simulink model "IEEE9_case"  (R2024b)
settings: Solver=FixedStepAuto  StartTime=0  StopTime=5  FixedStep=1e-7  RelTol=1e-3
values from neighbouring files (symbols this model uses):
  SG_D_1_D = 0.01056    [IEEE9_case_parameters.m]    (also in case1_parameters.m; case2_parameters.m; case3_parameters.m; case4_parameters.m)
  SG_D_1_EnableSaturation = 0    [IEEE9_case_parameters.m]    (also in case1_parameters.m; case2_parameters.m; case3_parameters.m; case4_parameters.m)
  SG_D_1_f0 = 60    [IEEE9_case_parameters.m]    (also in case1_parameters.m; case2_parameters.m; case3_parameters.m; case4_parameters.m)
  SG_D_1_H = 7.5    [IEEE9_case_parameters.m]    (also in case1_parameters.m; case2_parameters.m; case3_parameters.m; case4_parameters.m)
  SG_D_1_K_A = 20    [IEEE9_case_parameters.m]    (also in case1_parameters.m; case2_parameters.m; case3_parameters.m; case4_parameters.m)
  SG_D_1_K_E = 1.000000e+1    (= 10)    [IEEE9_case_parameters.m]    (also in case1_parameters.m; case2_parameters.m; case3_parameters.m; case4_parameters.m)
  SG_D_1_K_F = 2.363    [IEEE9_case_parameters.m]    (also in case1_parameters.m; case2_parameters.m; case3_parameters.m; case4_parameters.m)
  SG_D_1_K_s = 0.5    [IEEE9_case_parameters.m]    (also in case1_parameters.m = 5; case2_parameters.m = 5; case3_parameters.m = 5; case4_parameters.m = 5)
  SG_D_1_R_a = 0.001088    [IEEE9_case_parameters.m]    (also in case1_parameters.m; case2_parameters.m; case3_parameters.m; case4_parameters.m)
  SG_D_1_S_A = 1    [IEEE9_case_parameters.m]    (also in case1_parameters.m; case2_parameters.m; case3_parameters.m; case4_parameters.m)
  SG_D_1_S_B = 0.103    [IEEE9_case_parameters.m]    (also in case1_parameters.m; case2_parameters.m; case3_parameters.m; case4_parameters.m)
  SG_D_1_S_N = 10.659857    [IEEE9_case_parameters.m]    (also in case1_parameters.m; case2_parameters.m; case3_parameters.m; case4_parameters.m)
  SG_D_1_SpeedPara = 200    [IEEE9_case_parameters.m]    (also in case1_parameters.m; case2_parameters.m; case3_parameters.m; case4_parameters.m)
  SG_D_1_T_0 = 0.720173    [IEEE9_case_parameters.m]    (also in case1_parameters.m = 0.755522; case2_parameters.m = 0.808931; case3_parameters.m = 0.869402; case4_parameters.m = 0.729316)
  SG_D_1_T_1 = 0.3    [IEEE9_case_parameters.m]    (also in case1_parameters.m; case2_parameters.m; case3_parameters.m; case4_parameters.m)
  SG_D_1_T_2 = 0.05    [IEEE9_case_parameters.m]    (also in case1_parameters.m; case2_parameters.m; case3_parameters.m; case4_parameters.m)
  SG_D_1_T_3 = 0.02    [IEEE9_case_parameters.m]    (also in case1_parameters.m; case2_parameters.m; case3_parameters.m; case4_parameters.m)
  SG_D_1_T_4 = 0.005    [IEEE9_case_parameters.m]    (also in case1_parameters.m; case2_parameters.m; case3_parameters.m; case4_parameters.m)
  SG_D_1_T_A = 0.02    [IEEE9_case_parameters.m]    (also in case1_parameters.m; case2_parameters.m; case3_parameters.m; case4_parameters.m)
  SG_D_1_T_dd = 8.000000e+0    (= 8)    [IEEE9_case_parameters.m]    (also in case1_parameters.m; case2_parameters.m; case3_parameters.m; case4_parameters.m)
  SG_D_1_T_ddd = 0.04    [IEEE9_case_parameters.m]    (also in case1_parameters.m; case2_parameters.m; case3_parameters.m; case4_parameters.m)
  SG_D_1_T_E = 0.314    [IEEE9_case_parameters.m]    (also in case1_parameters.m; case2_parameters.m; case3_parameters.m; case4_parameters.m)
  SG_D_1_T_F = 0.35    [IEEE9_case_parameters.m]    (also in case1_parameters.m; case2_parameters.m; case3_parameters.m; case4_parameters.m)
  SG_D_1_T_qd = 0.8    [IEEE9_case_parameters.m]    (also in case1_parameters.m; case2_parameters.m; case3_parameters.m; case4_parameters.m)
  SG_D_1_T_qdd = 0.02    [IEEE9_case_parameters.m]    (also in case1_parameters.m; case2_parameters.m; case3_parameters.m; case4_parameters.m)
  SG_D_1_T_speed = 0.1    [IEEE9_case_parameters.m]    (also in case1_parameters.m = 200; case2_parameters.m = 200; case3_parameters.m = 200; case4_parameters.m = 200)
  SG_D_1_T_w = 0.5    [IEEE9_case_parameters.m]    (also in case1_parameters.m; case2_parameters.m; case3_parameters.m; case4_parameters.m)
  SG_D_1_V_ref = 1.990276    [IEEE9_case_parameters.m]    (also in case1_parameters.m = 2.042296; case2_parameters.m = 2.051388; case3_parameters.m = 2.089584; case4_parameters.m = 2.01845)
  SG_D_1_w_ref = 376.991118    [IEEE9_case_parameters.m]    (also in case1_parameters.m; case2_parameters.m; case3_parameters.m; case4_parameters.m)
  SG_D_1_wb = 6.000000e+1    (= 60)    [IEEE9_case_parameters.m]    (also in case1_parameters.m; case2_parameters.m; case3_parameters.m; case4_parameters.m)
  SG_D_1_x_d = 1.9    [IEEE9_case_parameters.m]    (also in case1_parameters.m; case2_parameters.m; case3_parameters.m; case4_parameters.m)
  SG_D_1_x_dd = 0.302    [IEEE9_case_parameters.m]    (also in case1_parameters.m; case2_parameters.m; case3_parameters.m; case4_parameters.m)
  SG_D_1_x_ddd = 0.204    [IEEE9_case_parameters.m]    (also in case1_parameters.m; case2_parameters.m; case3_parameters.m; case4_parameters.m)
  SG_D_1_x_l = 0.05    [IEEE9_case_parameters.m]    (also in case1_parameters.m; case2_parameters.m; case3_parameters.m; case4_parameters.m)
  SG_D_1_x_q = 1.3    [IEEE9_case_parameters.m]    (also in case1_parameters.m; case2_parameters.m; case3_parameters.m; case4_parameters.m)
  SG_D_1_x_qd = 0.5    [IEEE9_case_parameters.m]    (also in case1_parameters.m; case2_parameters.m; case3_parameters.m; case4_parameters.m)
  SG_D_1_x_qdd = 0.3    [IEEE9_case_parameters.m]    (also in case1_parameters.m; case2_parameters.m; case3_parameters.m; case4_parameters.m)
  SG_D_2_D = 0.02    [IEEE9_case_parameters.m]    (also in case1_parameters.m; case2_parameters.m; case3_parameters.m; case4_parameters.m)
  SG_D_2_EnableSaturation = 0    [IEEE9_case_parameters.m]    (also in case1_parameters.m; case2_parameters.m; case3_parameters.m; case4_parameters.m)
  SG_D_2_f0 = 60    [IEEE9_case_parameters.m]    (also in case1_parameters.m; case2_parameters.m; case3_parameters.m; case4_parameters.m)
  SG_D_2_H = 8.000000e+0    (= 8)    [IEEE9_case_parameters.m]    (also in case1_parameters.m; case2_parameters.m; case3_parameters.m; case4_parameters.m)
  SG_D_2_K_A = 20    [IEEE9_case_parameters.m]    (also in case1_parameters.m; case2_parameters.m; case3_parameters.m; case4_parameters.m)
  SG_D_2_K_E = 1.000000e+1    (= 10)    [IEEE9_case_parameters.m]    (also in case1_parameters.m; case2_parameters.m; case3_parameters.m; case4_parameters.m)
  SG_D_2_K_F = 2.363    [IEEE9_case_parameters.m]    (also in case1_parameters.m; case2_parameters.m; case3_parameters.m; case4_parameters.m)
  SG_D_2_K_s = 0.5    [IEEE9_case_parameters.m]    (also in case1_parameters.m = 4; case2_parameters.m = 4; case3_parameters.m = 4; case4_parameters.m = 4)
  SG_D_2_R_a = 0.001088    [IEEE9_case_parameters.m]    (also in case1_parameters.m; case2_parameters.m; case3_parameters.m; case4_parameters.m)
  SG_D_2_S_A = 1    [IEEE9_case_parameters.m]    (also in case1_parameters.m; case2_parameters.m; case3_parameters.m; case4_parameters.m)
  SG_D_2_S_B = 0.103    [IEEE9_case_parameters.m]    (also in case1_parameters.m; case2_parameters.m; case3_parameters.m; case4_parameters.m)
  SG_D_2_S_N = 10.659857    [IEEE9_case_parameters.m]    (also in case1_parameters.m; case2_parameters.m; case3_parameters.m; case4_parameters.m)
  SG_D_2_SpeedPara = 200    [IEEE9_case_parameters.m]    (also in case1_parameters.m; case2_parameters.m; case3_parameters.m; case4_parameters.m)
  SG_D_2_T_0 = 1.632913    [IEEE9_case_parameters.m]    (also in case1_parameters.m = 1.632925; case2_parameters.m = 1.632915; case3_parameters.m = 1.632914; case4_parameters.m = 1.632927)
  SG_D_2_T_1 = 0.2    [IEEE9_case_parameters.m]    (also in case1_parameters.m; case2_parameters.m; case3_parameters.m; case4_parameters.m)
  SG_D_2_T_2 = 0.05    [IEEE9_case_parameters.m]    (also in case1_parameters.m; case2_parameters.m; case3_parameters.m; case4_parameters.m)
  SG_D_2_T_3 = 0.02    [IEEE9_case_parameters.m]    (also in case1_parameters.m; case2_parameters.m; case3_parameters.m; case4_parameters.m)
  SG_D_2_T_4 = 0.005    [IEEE9_case_parameters.m]    (also in case1_parameters.m; case2_parameters.m; case3_parameters.m; case4_parameters.m)
  SG_D_2_T_A = 0.02    [IEEE9_case_parameters.m]    (also in case1_parameters.m; case2_parameters.m; case3_parameters.m; case4_parameters.m)
  SG_D_2_T_dd = 7.9    [IEEE9_case_parameters.m]    (also in case1_parameters.m; case2_parameters.m; case3_parameters.m; case4_parameters.m)
  SG_D_2_T_ddd = 0.04    [IEEE9_case_parameters.m]    (also in case1_parameters.m; case2_parameters.m; case3_parameters.m; case4_parameters.m)
  SG_D_2_T_E = 0.314    [IEEE9_case_parameters.m]    (also in case1_parameters.m; case2_parameters.m; case3_parameters.m; case4_parameters.m)
  SG_D_2_T_F = 0.35    [IEEE9_case_parameters.m]    (also in case1_parameters.m; case2_parameters.m; case3_parameters.m; case4_parameters.m)
  SG_D_2_T_qd = 0.8    [IEEE9_case_parameters.m]    (also in case1_parameters.m; case2_parameters.m; case3_parameters.m; case4_parameters.m)
  SG_D_2_T_qdd = 0.015    [IEEE9_case_parameters.m]    (also in case1_parameters.m; case2_parameters.m; case3_parameters.m; case4_parameters.m)
  SG_D_2_T_speed = 0.1    [IEEE9_case_parameters.m]    (also in case1_parameters.m = 150; case2_parameters.m = 150; case3_parameters.m = 150; case4_parameters.m = 150)
  SG_D_2_T_w = 0.35    [IEEE9_case_parameters.m]    (also in case1_parameters.m; case2_parameters.m; case3_parameters.m; case4_parameters.m)
  SG_D_2_V_ref = 2.58547    [IEEE9_case_parameters.m]    (also in case1_parameters.m = 2.597896; case2_parameters.m = 2.587136; case3_parameters.m = 2.586042; case4_parameters.m = 2.599679)
  SG_D_2_w_ref = 376.991118    [IEEE9_case_parameters.m]    (also in case1_parameters.m; case2_parameters.m; case3_parameters.m; case4_parameters.m)
  SG_D_2_wb = 6.000000e+1    (= 60)    [IEEE9_case_parameters.m]    (also in case1_parameters.m; case2_parameters.m; case3_parameters.m; case4_parameters.m)
  SG_D_2_x_d = 1.8    [IEEE9_case_parameters.m]    (also in case1_parameters.m; case2_parameters.m; case3_parameters.m; case4_parameters.m)
  SG_D_2_x_dd = 0.302    [IEEE9_case_parameters.m]    (also in case1_parameters.m; case2_parameters.m; case3_parameters.m; case4_parameters.m)
  SG_D_2_x_ddd = 0.204    [IEEE9_case_parameters.m]    (also in case1_parameters.m; case2_parameters.m; case3_parameters.m; case4_parameters.m)
  SG_D_2_x_l = 0.05    [IEEE9_case_parameters.m]    (also in case1_parameters.m; case2_parameters.m; case3_parameters.m; case4_parameters.m)
  SG_D_2_x_q = 1.25    [IEEE9_case_parameters.m]    (also in case1_parameters.m; case2_parameters.m; case3_parameters.m; case4_parameters.m)
  SG_D_2_x_qd = 0.5    [IEEE9_case_parameters.m]    (also in case1_parameters.m; case2_parameters.m; case3_parameters.m; case4_parameters.m)
  SG_D_2_x_qdd = 0.3    [IEEE9_case_parameters.m]    (also in case1_parameters.m; case2_parameters.m; case3_parameters.m; case4_parameters.m)
  SG_D_3_D = 0.02    [IEEE9_case_parameters.m]    (also in case1_parameters.m; case2_parameters.m; case3_parameters.m; case4_parameters.m)
  SG_D_3_EnableSaturation = 0    [IEEE9_case_parameters.m]    (also in case1_parameters.m; case2_parameters.m; case3_parameters.m; case4_parameters.m)
  SG_D_3_f0 = 60    [IEEE9_case_parameters.m]    (also in case1_parameters.m; case2_parameters.m; case3_parameters.m; case4_parameters.m)
  SG_D_3_H = 7.7    [IEEE9_case_parameters.m]    (also in case1_parameters.m; case2_parameters.m; case3_parameters.m; case4_parameters.m)
  SG_D_3_K_A = 20    [IEEE9_case_parameters.m]    (also in case1_parameters.m; case2_parameters.m; case3_parameters.m; case4_parameters.m)
  SG_D_3_K_E = 1.000000e+1    (= 10)    [IEEE9_case_parameters.m]    (also in case1_parameters.m; case2_parameters.m; case3_parameters.m; case4_parameters.m)
  SG_D_3_K_F = 2.363    [IEEE9_case_parameters.m]    (also in case1_parameters.m; case2_parameters.m; case3_parameters.m; case4_parameters.m)
  SG_D_3_K_s = 0.2    [IEEE9_case_parameters.m]    (also in case1_parameters.m = 2; case2_parameters.m = 2; case3_parameters.m = 2; case4_parameters.m = 2)
  SG_D_3_R_a = 0.001088    [IEEE9_case_parameters.m]    (also in case1_parameters.m; case2_parameters.m; case3_parameters.m; case4_parameters.m)
  SG_D_3_S_A = 1    [IEEE9_case_parameters.m]    (also in case1_parameters.m; case2_parameters.m; case3_parameters.m; case4_parameters.m)
  SG_D_3_S_B = 0.103    [IEEE9_case_parameters.m]    (also in case1_parameters.m; case2_parameters.m; case3_parameters.m; case4_parameters.m)
  SG_D_3_S_N = 10.659857    [IEEE9_case_parameters.m]    (also in case1_parameters.m; case2_parameters.m; case3_parameters.m; case4_parameters.m)
  SG_D_3_SpeedPara = 200    [IEEE9_case_parameters.m]    (also in case1_parameters.m; case2_parameters.m; case3_parameters.m; case4_parameters.m)
  SG_D_3_T_0 = 0.850788    [IEEE9_case_parameters.m]    (also in case1_parameters.m = 0.850786; case2_parameters.m = 0.850787; case3_parameters.m; case4_parameters.m = 0.850786)
  SG_D_3_T_1 = 0.2    [IEEE9_case_parameters.m]    (also in case1_parameters.m; case2_parameters.m; case3_parameters.m; case4_parameters.m)
  SG_D_3_T_2 = 0.05    [IEEE9_case_parameters.m]    (also in case1_parameters.m; case2_parameters.m; case3_parameters.m; case4_parameters.m)
  SG_D_3_T_3 = 0.02    [IEEE9_case_parameters.m]    (also in case1_parameters.m; case2_parameters.m; case3_parameters.m; case4_parameters.m)
  SG_D_3_T_4 = 0.005    [IEEE9_case_parameters.m]    (also in case1_parameters.m; case2_parameters.m; case3_parameters.m; case4_parameters.m)
  SG_D_3_T_A = 0.02    [IEEE9_case_parameters.m]    (also in case1_parameters.m; case2_parameters.m; case3_parameters.m; case4_parameters.m)
  SG_D_3_T_dd = 8.1    [IEEE9_case_parameters.m]    (also in case1_parameters.m; case2_parameters.m; case3_parameters.m; case4_parameters.m)
  SG_D_3_T_ddd = 0.04    [IEEE9_case_parameters.m]    (also in case1_parameters.m; case2_parameters.m; case3_parameters.m; case4_parameters.m)
  SG_D_3_T_E = 0.314    [IEEE9_case_parameters.m]    (also in case1_parameters.m; case2_parameters.m; case3_parameters.m; case4_parameters.m)
  SG_D_3_T_F = 0.35    [IEEE9_case_parameters.m]    (also in case1_parameters.m; case2_parameters.m; case3_parameters.m; case4_parameters.m)
  SG_D_3_T_qd = 0.8    [IEEE9_case_parameters.m]    (also in case1_parameters.m; case2_parameters.m; case3_parameters.m; case4_parameters.m)
  SG_D_3_T_qdd = 0.015    [IEEE9_case_parameters.m]    (also in case1_parameters.m; case2_parameters.m; case3_parameters.m; case4_parameters.m)
  SG_D_3_T_speed = 0.1    [IEEE9_case_parameters.m]    (also in case1_parameters.m = 180; case2_parameters.m = 180; case3_parameters.m = 180; case4_parameters.m = 180)
  SG_D_3_T_w = 0.4    [IEEE9_case_parameters.m]    (also in case1_parameters.m; case2_parameters.m; case3_parameters.m; case4_parameters.m)
  SG_D_3_V_ref = 1.892727    [IEEE9_case_parameters.m]    (also in case1_parameters.m = 1.906439; case2_parameters.m = 1.895535; case3_parameters.m = 1.892105; case4_parameters.m = 1.906598)
  SG_D_3_w_ref = 376.991118    [IEEE9_case_parameters.m]    (also in case1_parameters.m; case2_parameters.m; case3_parameters.m; case4_parameters.m)
  SG_D_3_wb = 6.000000e+1    (= 60)    [IEEE9_case_parameters.m]    (also in case1_parameters.m; case2_parameters.m; case3_parameters.m; case4_parameters.m)
  SG_D_3_x_d = 1.85    [IEEE9_case_parameters.m]    (also in case1_parameters.m; case2_parameters.m; case3_parameters.m; case4_parameters.m)
  SG_D_3_x_dd = 0.302    [IEEE9_case_parameters.m]    (also in case1_parameters.m; case2_parameters.m; case3_parameters.m; case4_parameters.m)
  SG_D_3_x_ddd = 0.204    [IEEE9_case_parameters.m]    (also in case1_parameters.m; case2_parameters.m; case3_parameters.m; case4_parameters.m)
  SG_D_3_x_l = 0.05    [IEEE9_case_parameters.m]    (also in case1_parameters.m; case2_parameters.m; case3_parameters.m; case4_parameters.m)
  SG_D_3_x_q = 1.2    [IEEE9_case_parameters.m]    (also in case1_parameters.m; case2_parameters.m; case3_parameters.m; case4_parameters.m)
  SG_D_3_x_qd = 0.5    [IEEE9_case_parameters.m]    (also in case1_parameters.m; case2_parameters.m; case3_parameters.m; case4_parameters.m)
  SG_D_3_x_qdd = 0.3    [IEEE9_case_parameters.m]    (also in case1_parameters.m; case2_parameters.m; case3_parameters.m; case4_parameters.m)
(part 4 of 12)

== system IEEE9_case/AC_1/d_vq_bus_4_block ==
  note: d_vq_bus_4 in IEEE9_case
      | $2257.43184689087\,\mathrm{iq}_{\mathrm{bus},4}-376.991118430775\,\mathrm{vd}_{\mathrm{bus},4}$
      | Automatically generated on 2025-11-01 08:50:43 .
  Alge_iq_bus_4_34632 : Inport
  State_vd_bus_4_b9421 : Inport  Port=2
  Constant_2257.43184689087_9b500 : Constant  Value=2257.43184689087
  Constant_376.991118430775_1fcb2 : Constant  Value=376.991118430775
  Product_358d4 : Product
  Product_fc33b : Product
  Subtract_b30ea : Sum  Inputs=+-
  Blockout_d_vq_bus_4_1d44a : Outport
  wires:
  Constant_2257.43184689087_9b500/1 -> Product_fc33b/1
  Constant_376.991118430775_1fcb2/1 -> Product_358d4/1
  Alge_iq_bus_4_34632/1 -> Product_fc33b/2
  State_vd_bus_4_b9421/1 -> Product_358d4/2
  Product_fc33b/1 -> Subtract_b30ea/1
  Product_358d4/1 -> Subtract_b30ea/2
  Subtract_b30ea/1 -> Blockout_d_vq_bus_4_1d44a/1

== system IEEE9_case/AC_1/d_vq_bus_5_block ==
  note: d_vq_bus_5 in IEEE9_case
      | $1461.2058853906\,\mathrm{iq}_{\mathrm{bus},5}-376.991118430775\,\mathrm{vd}_{\mathrm{bus},5}$
      | Automatically generated on 2025-11-01 08:50:45 .
  Alge_iq_bus_5_29d6a : Inport
  State_vd_bus_5_4af70 : Inport  Port=2
  Constant_1461.2058853906_07e73 : Constant  Value=1461.2058853906
  Constant_376.991118430775_33df4 : Constant  Value=376.991118430775
  Product_65bd2 : Product
  Product_9d57c : Product
  Subtract_81b72 : Sum  Inputs=+-
  Blockout_d_vq_bus_5_7aa33 : Outport
  wires:
  Constant_1461.2058853906_07e73/1 -> Product_9d57c/1
  Constant_376.991118430775_33df4/1 -> Product_65bd2/1
  Alge_iq_bus_5_29d6a/1 -> Product_9d57c/2
  State_vd_bus_5_4af70/1 -> Product_65bd2/2
  Product_9d57c/1 -> Subtract_81b72/1
  Product_65bd2/1 -> Subtract_81b72/2
  Subtract_81b72/1 -> Blockout_d_vq_bus_5_7aa33/1

== system IEEE9_case/AC_1/d_vq_bus_6_block ==
  note: d_vq_bus_6 in IEEE9_case
      | $1329.77466818616\,\mathrm{iq}_{\mathrm{bus},6}-376.991118430775\,\mathrm{vd}_{\mathrm{bus},6}$
      | Automatically generated on 2025-11-01 08:50:46 .
  Alge_iq_bus_6_36995 : Inport
  State_vd_bus_6_2a50c : Inport  Port=2
  Constant_1329.77466818616_5a7f1 : Constant  Value=1329.77466818616
  Constant_376.991118430775_38292 : Constant  Value=376.991118430775
  Product_76386 : Product
  Product_c695d : Product
  Subtract_bdad2 : Sum  Inputs=+-
  Blockout_d_vq_bus_6_9f6d7 : Outport
  wires:
  Constant_1329.77466818616_5a7f1/1 -> Product_c695d/1
  Constant_376.991118430775_38292/1 -> Product_76386/1
  Alge_iq_bus_6_36995/1 -> Product_c695d/2
  State_vd_bus_6_2a50c/1 -> Product_76386/2
  Product_c695d/1 -> Subtract_bdad2/1
  Product_76386/1 -> Subtract_bdad2/2
  Subtract_bdad2/1 -> Blockout_d_vq_bus_6_9f6d7/1

== system IEEE9_case/AC_1/d_vq_bus_7_block ==
  note: d_vq_bus_7 in IEEE9_case
      | $2106.09563369148\,\mathrm{iq}_{\mathrm{bus},7}-376.991118430775\,\mathrm{vd}_{\mathrm{bus},7}$
      | Automatically generated on 2025-11-01 08:50:48 .
  Alge_iq_bus_7_41fff : Inport
  State_vd_bus_7_b9fb4 : Inport  Port=2
  Constant_2106.09563369148_aa07a : Constant  Value=2106.09563369148
  Constant_376.991118430775_3bd3b : Constant  Value=376.991118430775
  Product_da61b : Product
  Product_e198d : Product
  Subtract_1132c : Sum  Inputs=+-
  Blockout_d_vq_bus_7_ac7ae : Outport
  wires:
  Constant_2106.09563369148_aa07a/1 -> Product_da61b/1
  Product_e198d/1 -> Subtract_1132c/2
  Alge_iq_bus_7_41fff/1 -> Product_da61b/2
  Constant_376.991118430775_3bd3b/1 -> Product_e198d/1
  Subtract_1132c/1 -> Blockout_d_vq_bus_7_ac7ae/1
  State_vd_bus_7_b9fb4/1 -> Product_e198d/2
  Product_da61b/1 -> Subtract_1132c/1

== system IEEE9_case/AC_1/d_vq_bus_8_block ==
  note: d_vq_bus_8 in IEEE9_case
      | $1657.10381727813\,\mathrm{iq}_{\mathrm{bus},8}-376.991118430775\,\mathrm{vd}_{\mathrm{bus},8}$
      | Automatically generated on 2025-11-01 08:50:49 .
  Alge_iq_bus_8_0a88b : Inport
  State_vd_bus_8_f2f43 : Inport  Port=2
  Constant_1657.10381727813_a5f6c : Constant  Value=1657.10381727813
  Constant_376.991118430775_b67aa : Constant  Value=376.991118430775
  Product_4c969 : Product
  Product_d050f : Product
  Subtract_7cb53 : Sum  Inputs=+-
  Blockout_d_vq_bus_8_bbe49 : Outport
  wires:
  Constant_1657.10381727813_a5f6c/1 -> Product_d050f/1
  Constant_376.991118430775_b67aa/1 -> Product_4c969/1
  Alge_iq_bus_8_0a88b/1 -> Product_d050f/2
  State_vd_bus_8_f2f43/1 -> Product_4c969/2
  Product_d050f/1 -> Subtract_7cb53/1
  Product_4c969/1 -> Subtract_7cb53/2
  Subtract_7cb53/1 -> Blockout_d_vq_bus_8_bbe49/1

== system IEEE9_case/AC_1/d_vq_bus_9_block ==
  note: d_vq_bus_9 in IEEE9_case
      | $1564.27849971276\,\mathrm{iq}_{\mathrm{bus},9}-376.991118430775\,\mathrm{vd}_{\mathrm{bus},9}$
      | Automatically generated on 2025-11-01 08:50:51 .
  Alge_iq_bus_9_8c1c8 : Inport
  State_vd_bus_9_79c64 : Inport  Port=2
  Constant_1564.27849971276_55199 : Constant  Value=1564.27849971276
  Constant_376.991118430775_19f1a : Constant  Value=376.991118430775
  Product_10283 : Product
  Product_a9d4d : Product
  Subtract_84a22 : Sum  Inputs=+-
  Blockout_d_vq_bus_9_bd9e0 : Outport
  wires:
  Constant_1564.27849971276_55199/1 -> Product_a9d4d/1
  Constant_376.991118430775_19f1a/1 -> Product_10283/1
  Alge_iq_bus_9_8c1c8/1 -> Product_a9d4d/2
  State_vd_bus_9_79c64/1 -> Product_10283/2
  Product_a9d4d/1 -> Subtract_84a22/1
  Product_10283/1 -> Subtract_84a22/2
  Subtract_84a22/1 -> Blockout_d_vq_bus_9_bd9e0/1

== system IEEE9_case/AC_1/id_bus_1_block ==
  note: id_bus_1 in IEEE9_case
      | $\mathrm{id}_{\mathrm{SG},D,1}-\mathrm{id}_{\mathrm{line},1,4}$
      | Automatically generated on 2025-11-01 08:51:19 .
  Input_id_SG_D_1_af302 : Inport
  State_id_line_1_4_3f82b : Inport  Port=2
  Subtract_48044 : Sum  Inputs=+-
  Blockout_id_bus_1_1926f : Outport
  wires:
  Input_id_SG_D_1_af302/1 -> Subtract_48044/1
  State_id_line_1_4_3f82b/1 -> Subtract_48044/2
  Subtract_48044/1 -> Blockout_id_bus_1_1926f/1

== system IEEE9_case/AC_1/id_bus_2_block ==
  note: id_bus_2 in IEEE9_case
      | $\mathrm{id}_{\mathrm{SG},D,2}+\mathrm{id}_{\mathrm{line},8,2}$
      | Automatically generated on 2025-11-01 08:51:21 .
  Input_id_SG_D_2_61c78 : Inport
  State_id_line_8_2_3c453 : Inport  Port=2
  Add_51e54 : Sum
  Blockout_id_bus_2_b293f : Outport
  wires:
  Input_id_SG_D_2_61c78/1 -> Add_51e54/1
  State_id_line_8_2_3c453/1 -> Add_51e54/2
  Add_51e54/1 -> Blockout_id_bus_2_b293f/1

== system IEEE9_case/AC_1/id_bus_3_block ==
  note: id_bus_3 in IEEE9_case
      | $\mathrm{id}_{\mathrm{SG},D,3}-\mathrm{id}_{\mathrm{line},3,6}$
      | Automatically generated on 2025-11-01 08:51:24 .
  Input_id_SG_D_3_1023f : Inport
  State_id_line_3_6_dffa3 : Inport  Port=2
  Subtract_aa28f : Sum  Inputs=+-
  Blockout_id_bus_3_4fcdf : Outport
  wires:
  Input_id_SG_D_3_1023f/1 -> Subtract_aa28f/1
  State_id_line_3_6_dffa3/1 -> Subtract_aa28f/2
  Subtract_aa28f/1 -> Blockout_id_bus_3_4fcdf/1

== system IEEE9_case/AC_1/id_bus_4_block ==
  note: id_bus_4 in IEEE9_case
      | $\mathrm{id}_{\mathrm{line},1,4}-\mathrm{id}_{\mathrm{line},4,5}+\mathrm{id}_{\mathrm{line},9,4}$
      | Automatically generated on 2025-11-01 08:51:25 .
  State_id_line_1_4_529f6 : Inport
  State_id_line_4_5_a587b : Inport  Port=2
  State_id_line_9_4_59811 : Inport  Port=3
  Add_436a9 : Sum
  Subtract_b4aea : Sum  Inputs=+-
  Blockout_id_bus_4_81819 : Outport
  wires:
  State_id_line_9_4_59811/1 -> Add_436a9/2
  State_id_line_1_4_529f6/1 -> Subtract_b4aea/1
  State_id_line_4_5_a587b/1 -> Subtract_b4aea/2
  Subtract_b4aea/1 -> Add_436a9/1
  Add_436a9/1 -> Blockout_id_bus_4_81819/1

== system IEEE9_case/AC_1/id_bus_5_block ==
  note: id_bus_5 in IEEE9_case
      | $\mathrm{id}_{\mathrm{line},4,5}-\mathrm{id}_{\mathrm{load},5}-\mathrm{id}_{\mathrm{line},5,6}$
      | Automatically generated on 2025-11-01 08:51:27 .
  State_id_load_5_f3160 : Inport
  State_id_line_4_5_e8389 : Inport  Port=2
  State_id_line_5_6_04d6d : Inport  Port=3
  Add_0c2c7 : Sum
  Constant_-1_94f82 : Constant  Value=-1
  Product_57124 : Product
  Subtract_8e2c4 : Sum  Inputs=+-
  Blockout_id_bus_5_24227 : Outport
  wires:
  Subtract_8e2c4/1 -> Blockout_id_bus_5_24227/1
  State_id_line_4_5_e8389/1 -> Add_0c2c7/2
  Constant_-1_94f82/1 -> Product_57124/1
  Add_0c2c7/1 -> Subtract_8e2c4/1
  State_id_load_5_f3160/1 -> Product_57124/2
  Product_57124/1 -> Add_0c2c7/1
  State_id_line_5_6_04d6d/1 -> Subtract_8e2c4/2

== system IEEE9_case/AC_1/id_bus_6_block ==
  note: id_bus_6 in IEEE9_case
      | $\mathrm{id}_{\mathrm{line},3,6}+\mathrm{id}_{\mathrm{line},5,6}-\mathrm{id}_{\mathrm{line},6,7}$
      | Automatically generated on 2025-11-01 08:51:28 .
  State_id_line_3_6_c2f24 : Inport
  State_id_line_5_6_c1efc : Inport  Port=2
  State_id_line_6_7_daca9 : Inport  Port=3
  Add_d01d1 : Sum
  Subtract_763e8 : Sum  Inputs=+-
  Blockout_id_bus_6_c0a22 : Outport
  wires:
  State_id_line_6_7_daca9/1 -> Subtract_763e8/2
  State_id_line_3_6_c2f24/1 -> Add_d01d1/1
  State_id_line_5_6_c1efc/1 -> Add_d01d1/2
  Add_d01d1/1 -> Subtract_763e8/1
  Subtract_763e8/1 -> Blockout_id_bus_6_c0a22/1

== system IEEE9_case/AC_1/id_bus_7_block ==
  note: id_bus_7 in IEEE9_case
      | $\mathrm{id}_{\mathrm{line},6,7}-\mathrm{id}_{\mathrm{load},7}-\mathrm{id}_{\mathrm{line},7,8}$
      | Automatically generated on 2025-11-01 08:51:30 .
  State_id_load_7_e82b6 : Inport
  State_id_line_6_7_c0e22 : Inport  Port=2
  State_id_line_7_8_cc267 : Inport  Port=3
  Add_a82d2 : Sum
  Constant_-1_01d99 : Constant  Value=-1
  Product_6eb41 : Product
  Subtract_060fe : Sum  Inputs=+-
  Blockout_id_bus_7_6ffd7 : Outport
  wires:
  Subtract_060fe/1 -> Blockout_id_bus_7_6ffd7/1
  State_id_line_6_7_c0e22/1 -> Add_a82d2/2
  Constant_-1_01d99/1 -> Product_6eb41/1
  Add_a82d2/1 -> Subtract_060fe/1
  State_id_load_7_e82b6/1 -> Product_6eb41/2
  Product_6eb41/1 -> Add_a82d2/1
  State_id_line_7_8_cc267/1 -> Subtract_060fe/2

== system IEEE9_case/AC_1/id_bus_8_block ==
  note: id_bus_8 in IEEE9_case
      | $\mathrm{id}_{\mathrm{line},7,8}-\mathrm{id}_{\mathrm{line},8,2}-\mathrm{id}_{\mathrm{line},8,9}$
      | Automatically generated on 2025-11-01 08:51:31 .
  State_id_line_7_8_7df9d : Inport
  State_id_line_8_2_3341e : Inport  Port=2
  State_id_line_8_9_71460 : Inport  Port=3
  Subtract_5dc26 : Sum  Inputs=+-
  Subtract_5dd95 : Sum  Inputs=+-
  Blockout_id_bus_8_96b63 : Outport
  wires:
  State_id_line_8_9_71460/1 -> Subtract_5dc26/2
  State_id_line_7_8_7df9d/1 -> Subtract_5dd95/1
  State_id_line_8_2_3341e/1 -> Subtract_5dd95/2
  Subtract_5dd95/1 -> Subtract_5dc26/1
  Subtract_5dc26/1 -> Blockout_id_bus_8_96b63/1

== system IEEE9_case/AC_1/id_bus_9_block ==
  note: id_bus_9 in IEEE9_case
      | $\mathrm{id}_{\mathrm{line},8,9}-\mathrm{id}_{\mathrm{load},9}-\mathrm{id}_{\mathrm{line},9,4}$
      | Automatically generated on 2025-11-01 08:51:32 .
  State_id_load_9_2a277 : Inport
  State_id_line_8_9_39eb5 : Inport  Port=2
  State_id_line_9_4_cdab0 : Inport  Port=3
  Add_27471 : Sum
  Constant_-1_a4445 : Constant  Value=-1
  Product_86825 : Product
  Subtract_300e1 : Sum  Inputs=+-
  Blockout_id_bus_9_9113d : Outport
  wires:
  Subtract_300e1/1 -> Blockout_id_bus_9_9113d/1
  State_id_line_8_9_39eb5/1 -> Add_27471/2
  Constant_-1_a4445/1 -> Product_86825/1
  Add_27471/1 -> Subtract_300e1/1
  State_id_load_9_2a277/1 -> Product_86825/2
  Product_86825/1 -> Add_27471/1
  State_id_line_9_4_cdab0/1 -> Subtract_300e1/2

== system IEEE9_case/AC_1/iq_bus_1_block ==
  note: iq_bus_1 in IEEE9_case
      | $\mathrm{iq}_{\mathrm{SG},D,1}-\mathrm{iq}_{\mathrm{line},1,4}$
      | Automatically generated on 2025-11-01 08:51:19 .
  Input_iq_SG_D_1_4742e : Inport
  State_iq_line_1_4_ea68f : Inport  Port=2
  Subtract_db840 : Sum  Inputs=+-
  Blockout_iq_bus_1_a22e6 : Outport
  wires:
  Input_iq_SG_D_1_4742e/1 -> Subtract_db840/1
  State_iq_line_1_4_ea68f/1 -> Subtract_db840/2
  Subtract_db840/1 -> Blockout_iq_bus_1_a22e6/1

== system IEEE9_case/AC_1/iq_bus_2_block ==
  note: iq_bus_2 in IEEE9_case
      | $\mathrm{iq}_{\mathrm{SG},D,2}+\mathrm{iq}_{\mathrm{line},8,2}$
      | Automatically generated on 2025-11-01 08:51:22 .
  Input_iq_SG_D_2_0132f : Inport
  State_iq_line_8_2_dbe3b : Inport  Port=2
  Add_8c3a8 : Sum
  Blockout_iq_bus_2_7e5d3 : Outport
  wires:
  Input_iq_SG_D_2_0132f/1 -> Add_8c3a8/1
  State_iq_line_8_2_dbe3b/1 -> Add_8c3a8/2
  Add_8c3a8/1 -> Blockout_iq_bus_2_7e5d3/1

== system IEEE9_case/AC_1/iq_bus_3_block ==
  note: iq_bus_3 in IEEE9_case
      | $\mathrm{iq}_{\mathrm{SG},D,3}-\mathrm{iq}_{\mathrm{line},3,6}$
      | Automatically generated on 2025-11-01 08:51:24 .
  Input_iq_SG_D_3_bb505 : Inport
  State_iq_line_3_6_8c689 : Inport  Port=2
  Subtract_283a5 : Sum  Inputs=+-
  Blockout_iq_bus_3_2e2f8 : Outport
  wires:
  Input_iq_SG_D_3_bb505/1 -> Subtract_283a5/1
  State_iq_line_3_6_8c689/1 -> Subtract_283a5/2
  Subtract_283a5/1 -> Blockout_iq_bus_3_2e2f8/1

== system IEEE9_case/AC_1/iq_bus_4_block ==
  note: iq_bus_4 in IEEE9_case
      | $\mathrm{iq}_{\mathrm{line},1,4}-\mathrm{iq}_{\mathrm{line},4,5}+\mathrm{iq}_{\mathrm{line},9,4}$
      | Automatically generated on 2025-11-01 08:51:26 .
  State_iq_line_1_4_ad230 : Inport
  State_iq_line_4_5_86879 : Inport  Port=2
  State_iq_line_9_4_6d8cb : Inport  Port=3
  Add_e607c : Sum
  Subtract_70c7a : Sum  Inputs=+-
  Blockout_iq_bus_4_bba5d : Outport
  wires:
  State_iq_line_1_4_ad230/1 -> Subtract_70c7a/1
  State_iq_line_4_5_86879/1 -> Subtract_70c7a/2
  Subtract_70c7a/1 -> Add_e607c/1
  State_iq_line_9_4_6d8cb/1 -> Add_e607c/2
  Add_e607c/1 -> Blockout_iq_bus_4_bba5d/1

== system IEEE9_case/AC_1/iq_bus_5_block ==
  note: iq_bus_5 in IEEE9_case
      | $\mathrm{iq}_{\mathrm{line},4,5}-\mathrm{iq}_{\mathrm{load},5}-\mathrm{iq}_{\mathrm{line},5,6}$
      | Automatically generated on 2025-11-01 08:51:28 .
  State_iq_load_5_74a4d : Inport
  State_iq_line_4_5_0cb61 : Inport  Port=2
  State_iq_line_5_6_863ab : Inport  Port=3
  Add_5921b : Sum
  Constant_-1_83768 : Constant  Value=-1
  Product_975f6 : Product
  Subtract_2bfd8 : Sum  Inputs=+-
  Blockout_iq_bus_5_ca42e : Outport
  wires:
  Subtract_2bfd8/1 -> Blockout_iq_bus_5_ca42e/1
  State_iq_line_4_5_0cb61/1 -> Add_5921b/2
  Constant_-1_83768/1 -> Product_975f6/1
  State_iq_load_5_74a4d/1 -> Product_975f6/2
  Product_975f6/1 -> Add_5921b/1
  Add_5921b/1 -> Subtract_2bfd8/1
  State_iq_line_5_6_863ab/1 -> Subtract_2bfd8/2

== system IEEE9_case/AC_1/iq_bus_6_block ==
  note: iq_bus_6 in IEEE9_case
      | $\mathrm{iq}_{\mathrm{line},3,6}+\mathrm{iq}_{\mathrm{line},5,6}-\mathrm{iq}_{\mathrm{line},6,7}$
      | Automatically generated on 2025-11-01 08:51:29 .
  State_iq_line_3_6_b6d58 : Inport
  State_iq_line_5_6_aa0cd : Inport  Port=2
  State_iq_line_6_7_26089 : Inport  Port=3
  Add_a46ae : Sum
  Subtract_8afeb : Sum  Inputs=+-
  Blockout_iq_bus_6_857b2 : Outport
  wires:
  State_iq_line_3_6_b6d58/1 -> Add_a46ae/1
  State_iq_line_5_6_aa0cd/1 -> Add_a46ae/2
  Add_a46ae/1 -> Subtract_8afeb/1
  State_iq_line_6_7_26089/1 -> Subtract_8afeb/2
  Subtract_8afeb/1 -> Blockout_iq_bus_6_857b2/1

== system IEEE9_case/AC_1/iq_bus_7_block ==
  note: iq_bus_7 in IEEE9_case
      | $\mathrm{iq}_{\mathrm{line},6,7}-\mathrm{iq}_{\mathrm{load},7}-\mathrm{iq}_{\mathrm{line},7,8}$
      | Automatically generated on 2025-11-01 08:51:30 .
  State_iq_load_7_aef02 : Inport
  State_iq_line_6_7_e8477 : Inport  Port=2
  State_iq_line_7_8_380c1 : Inport  Port=3
  Add_af84e : Sum
  Constant_-1_169db : Constant  Value=-1
  Product_d2745 : Product
  Subtract_410e7 : Sum  Inputs=+-
  Blockout_iq_bus_7_2f8a2 : Outport
  wires:
  Subtract_410e7/1 -> Blockout_iq_bus_7_2f8a2/1
  State_iq_line_6_7_e8477/1 -> Add_af84e/2
  Constant_-1_169db/1 -> Product_d2745/1
  State_iq_load_7_aef02/1 -> Product_d2745/2
  Product_d2745/1 -> Add_af84e/1
  Add_af84e/1 -> Subtract_410e7/1
  State_iq_line_7_8_380c1/1 -> Subtract_410e7/2

== system IEEE9_case/AC_1/iq_bus_8_block ==
  note: iq_bus_8 in IEEE9_case
      | $\mathrm{iq}_{\mathrm{line},7,8}-\mathrm{iq}_{\mathrm{line},8,2}-\mathrm{iq}_{\mathrm{line},8,9}$
      | Automatically generated on 2025-11-01 08:51:32 .
  State_iq_line_7_8_d1eb2 : Inport
  State_iq_line_8_2_b7626 : Inport  Port=2
  State_iq_line_8_9_dde8d : Inport  Port=3
  Subtract_753be : Sum  Inputs=+-
  Subtract_98f60 : Sum  Inputs=+-
  Blockout_iq_bus_8_966d9 : Outport
  wires:
  State_iq_line_7_8_d1eb2/1 -> Subtract_98f60/1
  State_iq_line_8_2_b7626/1 -> Subtract_98f60/2
  Subtract_98f60/1 -> Subtract_753be/1
  State_iq_line_8_9_dde8d/1 -> Subtract_753be/2
  Subtract_753be/1 -> Blockout_iq_bus_8_966d9/1

== system IEEE9_case/AC_1/iq_bus_9_block ==
  note: iq_bus_9 in IEEE9_case
      | $\mathrm{iq}_{\mathrm{line},8,9}-\mathrm{iq}_{\mathrm{load},9}-\mathrm{iq}_{\mathrm{line},9,4}$
      | Automatically generated on 2025-11-01 08:51:33 .
  State_iq_load_9_c7015 : Inport
  State_iq_line_8_9_a5789 : Inport  Port=2
  State_iq_line_9_4_e3782 : Inport  Port=3
  Add_1de3e : Sum
  Constant_-1_ced50 : Constant  Value=-1
  Product_00029 : Product
  Subtract_fedab : Sum  Inputs=+-
  Blockout_iq_bus_9_298a2 : Outport
  wires:
  Subtract_fedab/1 -> Blockout_iq_bus_9_298a2/1
  State_iq_line_8_9_a5789/1 -> Add_1de3e/2
  Constant_-1_ced50/1 -> Product_00029/1
  State_iq_load_9_c7015/1 -> Product_00029/2
  Product_00029/1 -> Add_1de3e/1
  Add_1de3e/1 -> Subtract_fedab/1
  State_iq_line_9_4_e3782/1 -> Subtract_fedab/2

== system IEEE9_case/AC_1/vd_bus_1_out_block ==
  note: vd_bus_1_out in IEEE9_case
      | $\mathrm{vd}_{\mathrm{bus},1}$
      | Automatically generated on 2025-11-01 08:51:18 .
  State_vd_bus_1_74d9b : Inport
  Blockout_vd_bus_1_out_322ac : Outport
  wires:
  State_vd_bus_1_74d9b/1 -> Blockout_vd_bus_1_out_322ac/1

== system IEEE9_case/AC_1/vd_bus_2_out_block ==
  note: vd_bus_2_out in IEEE9_case
      | $\mathrm{vd}_{\mathrm{bus},2}$
      | Automatically generated on 2025-11-01 08:51:20 .
  State_vd_bus_2_cb137 : Inport
  Blockout_vd_bus_2_out_4b0bd : Outport
  wires:
  State_vd_bus_2_cb137/1 -> Blockout_vd_bus_2_out_4b0bd/1

== system IEEE9_case/AC_1/vd_bus_3_out_block ==
  note: vd_bus_3_out in IEEE9_case
      | $\mathrm{vd}_{\mathrm{bus},3}$
      | Automatically generated on 2025-11-01 08:51:23 .
  State_vd_bus_3_ac381 : Inport
  Blockout_vd_bus_3_out_d8755 : Outport
  wires:
  State_vd_bus_3_ac381/1 -> Blockout_vd_bus_3_out_d8755/1

== system IEEE9_case/AC_1/vq_bus_1_out_block ==
  note: vq_bus_1_out in IEEE9_case
      | $\mathrm{vq}_{\mathrm{bus},1}$
      | Automatically generated on 2025-11-01 08:51:18 .
  State_vq_bus_1_ae316 : Inport
  Blockout_vq_bus_1_out_2811e : Outport
  wires:
  State_vq_bus_1_ae316/1 -> Blockout_vq_bus_1_out_2811e/1

== system IEEE9_case/AC_1/vq_bus_2_out_block ==
  note: vq_bus_2_out in IEEE9_case
      | $\mathrm{vq}_{\mathrm{bus},2}$
      | Automatically generated on 2025-11-01 08:51:21 .
  State_vq_bus_2_ae5be : Inport
  Blockout_vq_bus_2_out_a1917 : Outport
  wires:
  State_vq_bus_2_ae5be/1 -> Blockout_vq_bus_2_out_a1917/1

== system IEEE9_case/AC_1/vq_bus_3_out_block ==
  note: vq_bus_3_out in IEEE9_case
      | $\mathrm{vq}_{\mathrm{bus},3}$
      | Automatically generated on 2025-11-01 08:51:23 .
  State_vq_bus_3_e6988 : Inport
  Blockout_vq_bus_3_out_d8ffc : Outport
  wires:
  State_vq_bus_3_e6988/1 -> Blockout_vq_bus_3_out_d8ffc/1

== system IEEE9_case/SG_D_1/T_e_SG_D_1_block ==
  note: T_e_SG_D_1 in IEEE9_case
      | $-\frac{\psi _{d,\mathrm{SG},D,1}\,\left(\psi _{q,\mathrm{SG},D,1}+\frac{\psi _{\mathrm{gq},\mathrm{SG},D,1}\,\left(x_{l}-x_{\mathrm{qdd}}\right)}{x_{l}-x_{\mathrm{qd}}}+\frac{\psi _{\mathrm{kq},\mathrm{SG},D,1}\,\left(x_{\mathrm{qd}}-x_{\mathrm{qdd}}\right)}{x_{l}-x_{\mathrm{qd}}}\right)}{x_{\mathrm{qdd}}}-\frac{\psi _{q,\mathrm{SG},D,1}\,\left(\frac{\psi _{\mathrm{1d},\mathrm{SG},D,1}\,\left(x_{\mathrm{dd}}-x_{\mathrm{ddd}}\right)}{x_{\mathrm{dd}}-x_{l}}-\psi _{d,\mathrm{SG},D,1}+\frac{\psi _{\mathrm{fd},\mathrm{SG},D,1}\,\left(x_{\mathrm{ddd}}-x_{l}\right)}{x_{\mathrm{dd}}-x_{l}}\right)}{x_{\mathrm{ddd}}}$
      | Automatically generated on 2025-11-01 08:48:20 .
  State_psi_d_SG_D_1_b48d8 : Inport
  State_psi_gq_SG_D_1_cded7 : Inport  Port=2
  State_psi_kq_SG_D_1_fce1a : Inport  Port=3
  State_psi_q_SG_D_1_125de : Inport  Port=4
  State_psi_q_SG_D_1_d8f2c : Inport  Port=5
  State_psi_1d_SG_D_1_22d02 : Inport  Port=6
  State_psi_d_SG_D_1_4849f : Inport  Port=7
  State_psi_fd_SG_D_1_a01cd : Inport  Port=8
  Add_00dea : Sum
  Add_13385 : Sum
  Add_2ca9d : Sum
  Add_3e6f8 : Sum
  Add_4acc2 : Sum
  Add_def3f : Sum
  Constant_-1_7cd7c : Constant  Value=-1
  Constant_-1_87de2 : Constant  Value=-1
  Constant_-1_a2826 : Constant  Value=-1
  Constant_-1_c783e : Constant  Value=-1
  Constant_-1_e74c3 : Constant  Value=-1
  Constant_x_dd_145e2 : Constant  Value=x_dd
  Constant_x_dd_27308 : Constant  Value=x_dd
  Constant_x_dd_d3c37 : Constant  Value=x_dd
  Constant_x_ddd_265a3 : Constant  Value=x_ddd
  Constant_x_ddd_2c9ce : Constant  Value=x_ddd
  Constant_x_ddd_aedfc : Constant  Value=x_ddd
  Constant_x_l_16a1c : Constant  Value=x_l
  Constant_x_l_38b79 : Constant  Value=x_l
  Constant_x_l_54c07 : Constant  Value=x_l
  Constant_x_l_6b6d9 : Constant  Value=x_l
  Constant_x_l_bb9d0 : Constant  Value=x_l
  Constant_x_l_c1d1d : Constant  Value=x_l
  Constant_x_qd_0598e : Constant  Value=x_qd
  Constant_x_qd_07235 : Constant  Value=x_qd
  Constant_x_qd_5a95c : Constant  Value=x_qd
  Constant_x_qdd_28c2a : Constant  Value=x_qdd
  Constant_x_qdd_43547 : Constant  Value=x_qdd
  Constant_x_qdd_bb72c : Constant  Value=x_qdd
  Divide_46449 : Product  Inputs=*/
  Divide_8674b : Product  Inputs=*/
  Divide_a32b2 : Product  Inputs=*/
  Divide_a7ba8 : Product  Inputs=*/
  Divide_ca26b : Product  Inputs=*/
  Divide_de1c1 : Product  Inputs=*/
  Product_7ec3f : Product
  Product_844df : Product
  Product_8df6f : Product
  Product_90535 : Product
  Product_9a007 : Product
  Product_a1923 : Product
  Product_b680a : Product
  Product_bb1b4 : Product
  Product_d3c92 : Product
  Product_edbef : Product
  Product_faa1a : Product
  Subtract_21db0 : Sum  Inputs=+-
  Subtract_4edb7 : Sum  Inputs=+-
  Subtract_6846c : Sum  Inputs=+-
  Subtract_7b57c : Sum  Inputs=+-
  Subtract_7e966 : Sum  Inputs=+-
  Subtract_b3a00 : Sum  Inputs=+-
  Subtract_f2908 : Sum  Inputs=+-
  Blockout_T_e_SG_D_1_44096 : Outport
  wires:
  Product_edbef/1 -> Divide_46449/1
  Product_844df/1 -> Add_def3f/1
  Divide_46449/1 -> Subtract_7e966/1
  Constant_-1_7cd7c/1 -> Product_844df/1
  Constant_x_l_38b79/1 -> Product_844df/2
  Constant_x_qdd_28c2a/1 -> Add_def3f/2
  Constant_x_qd_5a95c/1 -> Subtract_b3a00/1
  Constant_-1_c783e/1 -> Product_d3c92/1
  Constant_x_qdd_bb72c/1 -> Divide_a7ba8/2
  Constant_x_qdd_43547/1 -> Subtract_b3a00/2
  State_psi_q_SG_D_1_d8f2c/1 -> Product_7ec3f/1
  Constant_x_dd_27308/1 -> Subtract_7b57c/1
  Constant_x_l_54c07/1 -> Product_d3c92/2
  Subtract_7b57c/1 -> Product_b680a/2
  Constant_-1_87de2/1 -> Product_a1923/1
  Constant_x_l_c1d1d/1 -> Product_a1923/2
  Subtract_21db0/1 -> Product_7ec3f/2
  State_psi_q_SG_D_1_125de/1 -> Add_13385/2
  Constant_-1_e74c3/1 -> Product_9a007/1
  State_psi_1d_SG_D_1_22d02/1 -> Product_9a007/2
  Constant_x_ddd_aedfc/1 -> Subtract_7b57c/2
  State_psi_gq_SG_D_1_cded7/1 -> Product_edbef/1
  Add_def3f/1 -> Product_edbef/2
  Product_d3c92/1 -> Add_4acc2/1
  Product_90535/1 -> Product_bb1b4/1
  Constant_x_qd_07235/1 -> Add_4acc2/2
  Product_b680a/1 -> Divide_ca26b/1
  State_psi_kq_SG_D_1_fce1a/1 -> Product_faa1a/1
  Add_4acc2/1 -> Divide_46449/2
  Subtract_b3a00/1 -> Product_faa1a/2
  Product_a1923/1 -> Add_3e6f8/1
  Constant_x_qd_0598e/1 -> Add_3e6f8/2
  Product_faa1a/1 -> Divide_8674b/1
  Product_9a007/1 -> Product_b680a/1
  Constant_x_dd_145e2/1 -> Subtract_4edb7/1
  Constant_x_l_16a1c/1 -> Subtract_4edb7/2
  Constant_x_ddd_2c9ce/1 -> Subtract_f2908/1
  Product_7ec3f/1 -> Divide_a32b2/1
  Constant_x_l_bb9d0/1 -> Subtract_f2908/2
  Divide_a7ba8/1 -> Add_2ca9d/1
  Product_bb1b4/1 -> Divide_a7ba8/1
  Add_3e6f8/1 -> Divide_8674b/2
  Subtract_7e966/1 -> Add_13385/1
  Divide_8674b/1 -> Subtract_7e966/2
  Subtract_4edb7/1 -> Divide_ca26b/2
  State_psi_fd_SG_D_1_a01cd/1 -> Product_8df6f/1
  Constant_x_ddd_265a3/1 -> Divide_a32b2/2
  Subtract_f2908/1 -> Product_8df6f/2
  Constant_x_dd_d3c37/1 -> Subtract_6846c/1
  Constant_x_l_6b6d9/1 -> Subtract_6846c/2
  Divide_ca26b/1 -> Add_00dea/1
  Add_00dea/1 -> Subtract_21db0/1
  State_psi_d_SG_D_1_4849f/1 -> Add_00dea/2
  Product_8df6f/1 -> Divide_de1c1/1
  Subtract_6846c/1 -> Divide_de1c1/2
  Constant_-1_a2826/1 -> Product_90535/1
  State_psi_d_SG_D_1_b48d8/1 -> Product_90535/2
  Divide_de1c1/1 -> Subtract_21db0/2
  Add_13385/1 -> Product_bb1b4/2
  Divide_a32b2/1 -> Add_2ca9d/2
  Add_2ca9d/1 -> Blockout_T_e_SG_D_1_44096/1

== system IEEE9_case/SG_D_1/d_E_fd_SG_D_1_block ==
  note: d_E_fd_SG_D_1 in IEEE9_case
      | $\frac{V_{f,\mathrm{SG},D,1}-E_{\mathrm{fd},\mathrm{SG},D,1}\,K_{E}}{T_{E}}$
      | Automatically generated on 2025-11-01 08:48:03 .
  State_E_fd_SG_D_1_4ae7b : Inport
  State_V_f_SG_D_1_4d4c3 : Inport  Port=2
  Add_f4241 : Sum
  Constant_-1_2b163 : Constant  Value=-1
  Constant_K_E_3a206 : Constant  Value=K_E
  Constant_T_E_a46f0 : Constant  Value=T_E
  Divide_e0173 : Product  Inputs=*/
  Product_33762 : Product
  Product_b347f : Product
  Blockout_d_E_fd_SG_D_1_f9109 : Outport
  wires:
  Add_f4241/1 -> Divide_e0173/1
  Constant_-1_2b163/1 -> Product_33762/1
  State_E_fd_SG_D_1_4ae7b/1 -> Product_33762/2
  Product_33762/1 -> Product_b347f/1
  Constant_K_E_3a206/1 -> Product_b347f/2
  Product_b347f/1 -> Add_f4241/1
  Constant_T_E_a46f0/1 -> Divide_e0173/2
  State_V_f_SG_D_1_4d4c3/1 -> Add_f4241/2
  Divide_e0173/1 -> Blockout_d_E_fd_SG_D_1_f9109/1

== system IEEE9_case/SG_D_1/d_Px_1_SG_D_1_block ==
  note: d_Px_1_SG_D_1 in IEEE9_case
      | $\frac{w_{\mathrm{SG},D,1}-2\,\pi \,f_{0}}{T_{w}}-\frac{\mathrm{Px}_{1,\mathrm{SG},D,1}}{T_{w}}$
      | Automatically generated on 2025-11-01 08:48:04 .
  State_Px_1_SG_D_1_568ef : Inport
  State_w_SG_D_1_bae23 : Inport  Port=2
  Add_b0cdc : Sum
  Add_c7216 : Sum
  Constant_-1_ba5cd : Constant  Value=-1
  Constant_-2.0_674f8 : Constant  Value=-2.0
  Constant_T_w_46794 : Constant  Value=T_w
  Constant_T_w_bf8b9 : Constant  Value=T_w
  Constant_f0_b453c : Constant  Value=f0
  Constant_pi_b6898 : Constant  Value=pi
  Divide_229a2 : Product  Inputs=*/
  Divide_806a3 : Product  Inputs=*/
  Product_25483 : Product
  Product_717d3 : Product
  Product_79b9f : Product
  Blockout_d_Px_1_SG_D_1_5306e : Outport
  wires:
  Add_c7216/1 -> Blockout_d_Px_1_SG_D_1_5306e/1
  Constant_-2.0_674f8/1 -> Product_79b9f/1
  Product_25483/1 -> Divide_806a3/1
  State_w_SG_D_1_bae23/1 -> Add_b0cdc/2
  Constant_-1_ba5cd/1 -> Product_25483/1
  Constant_f0_b453c/1 -> Product_717d3/2
  Constant_pi_b6898/1 -> Product_79b9f/2
  Product_717d3/1 -> Add_b0cdc/1
  Product_79b9f/1 -> Product_717d3/1
  State_Px_1_SG_D_1_568ef/1 -> Product_25483/2
  Constant_T_w_46794/1 -> Divide_806a3/2
  Add_b0cdc/1 -> Divide_229a2/1
  Constant_T_w_bf8b9/1 -> Divide_229a2/2
  Divide_806a3/1 -> Add_c7216/1
  Divide_229a2/1 -> Add_c7216/2

== system IEEE9_case/SG_D_1/d_Px_2_SG_D_1_block ==
  note: d_Px_2_SG_D_1 in IEEE9_case
      | $\frac{\mathrm{Px}_{1,\mathrm{SG},D,1}-T_{2}\,\left(\frac{\mathrm{Px}_{1,\mathrm{SG},D,1}}{T_{w}}-\frac{w_{\mathrm{SG},D,1}-2\,\pi \,f_{0}}{T_{w}}\right)}{T_{1}}-\frac{\mathrm{Px}_{2,\mathrm{SG},D,1}}{T_{1}}$
      | Automatically generated on 2025-11-01 08:48:06 .
  State_Px_2_SG_D_1_c858b : Inport
  State_Px_1_SG_D_1_e7112 : Inport  Port=2
  State_Px_1_SG_D_1_31a86 : Inport  Port=3
  State_w_SG_D_1_fb742 : Inport  Port=4
  Add_b4878 : Sum
  Add_b7c78 : Sum
  Add_cf61d : Sum
  Add_ee85f : Sum
  Constant_-1_16318 : Constant  Value=-1
  Constant_-1_1c1af : Constant  Value=-1
  Constant_-2.0_2c114 : Constant  Value=-2.0
  Constant_T_1_1e672 : Constant  Value=T_1
  Constant_T_1_cc06b : Constant  Value=T_1
  Constant_T_2_9505b : Constant  Value=T_2
  Constant_T_w_26f40 : Constant  Value=T_w
  Constant_T_w_cded3 : Constant  Value=T_w
  Constant_f0_cd281 : Constant  Value=f0
  Constant_pi_d69eb : Constant  Value=pi
  Divide_1f3a5 : Product  Inputs=*/
  Divide_59115 : Product  Inputs=*/
  Divide_9810d : Product  Inputs=*/
  Divide_cb163 : Product  Inputs=*/
  Product_258e5 : Product
  Product_ab3b1 : Product
  Product_bc4a3 : Product
  Product_d0c9c : Product
  Product_ea409 : Product
  Blockout_d_Px_2_SG_D_1_88157 : Outport
  wires:
  Constant_-2.0_2c114/1 -> Product_bc4a3/1
  State_w_SG_D_1_fb742/1 -> Add_b7c78/2
  Constant_f0_cd281/1 -> Product_ea409/2
  Constant_pi_d69eb/1 -> Product_bc4a3/2
  Add_cf61d/1 -> Product_258e5/2
  Product_ea409/1 -> Add_b7c78/1
  Divide_9810d/1 -> Add_cf61d/1
  Product_bc4a3/1 -> Product_ea409/1
  Constant_T_w_cded3/1 -> Divide_9810d/2
  Constant_-1_16318/1 -> Product_ab3b1/1
  State_Px_1_SG_D_1_31a86/1 -> Product_ab3b1/2
  Divide_1f3a5/1 -> Add_ee85f/1
  Product_ab3b1/1 -> Divide_9810d/1
  Add_b7c78/1 -> Divide_59115/1
  Constant_T_w_26f40/1 -> Divide_59115/2
  Divide_59115/1 -> Add_cf61d/2
  Constant_T_2_9505b/1 -> Product_258e5/1
  Constant_-1_1c1af/1 -> Product_d0c9c/1
  State_Px_2_SG_D_1_c858b/1 -> Product_d0c9c/2
  State_Px_1_SG_D_1_e7112/1 -> Add_b4878/1
  Product_258e5/1 -> Add_b4878/2
  Add_b4878/1 -> Divide_cb163/1
  Product_d0c9c/1 -> Divide_1f3a5/1
  Constant_T_1_1e672/1 -> Divide_1f3a5/2
  Constant_T_1_cc06b/1 -> Divide_cb163/2
  Divide_cb163/1 -> Add_ee85f/2
  Add_ee85f/1 -> Blockout_d_Px_2_SG_D_1_88157/1

== system IEEE9_case/SG_D_1/d_Px_3_SG_D_1_block ==
  note: d_Px_3_SG_D_1 in IEEE9_case
      | $\frac{\mathrm{Px}_{2,\mathrm{SG},D,1}+T_{4}\,\left(\frac{\mathrm{Px}_{1,\mathrm{SG},D,1}-T_{2}\,\left(\frac{\mathrm{Px}_{1,\mathrm{SG},D,1}}{T_{w}}-\frac{w_{\mathrm{SG},D,1}-2\,\pi \,f_{0}}{T_{w}}\right)}{T_{1}}-\frac{\mathrm{Px}_{2,\mathrm{SG},D,1}}{T_{1}}\right)}{T_{3}}-\frac{\mathrm{Px}_{3,\mathrm{SG},D,1}}{T_{3}}$
      | Automatically generated on 2025-11-01 08:48:08 .
  State_Px_3_SG_D_1_17088 : Inport
  State_Px_2_SG_D_1_8d556 : Inport  Port=2
  State_Px_2_SG_D_1_a6db1 : Inport  Port=3
  State_Px_1_SG_D_1_a9a67 : Inport  Port=4
  State_Px_1_SG_D_1_15fdf : Inport  Port=5
  State_w_SG_D_1_3e7b9 : Inport  Port=6
  Add_3e2d0 : Sum
  Add_5625b : Sum
  Add_8be64 : Sum
  Add_a5a7f : Sum
  Add_ae2ce : Sum
  Add_ee9ea : Sum
  Constant_-1_4b8fe : Constant  Value=-1
  Constant_-1_6b6a5 : Constant  Value=-1
  Constant_-1_78b1b : Constant  Value=-1
  Constant_-2.0_88e6c : Constant  Value=-2.0
  Constant_T_1_5adde : Constant  Value=T_1
  Constant_T_1_cb6f1 : Constant  Value=T_1
  Constant_T_2_9e5a4 : Constant  Value=T_2
  Constant_T_3_8bbd7 : Constant  Value=T_3
  Constant_T_3_c6588 : Constant  Value=T_3
  Constant_T_4_0db6e : Constant  Value=T_4
  Constant_T_w_17b7c : Constant  Value=T_w
  Constant_T_w_ae441 : Constant  Value=T_w
  Constant_f0_8479a : Constant  Value=f0
  Constant_pi_eb74e : Constant  Value=pi
  Divide_0b283 : Product  Inputs=*/
  Divide_2beb5 : Product  Inputs=*/
  Divide_63b10 : Product  Inputs=*/
  Divide_b4ce1 : Product  Inputs=*/
  Divide_c2e41 : Product  Inputs=*/
  Divide_cb6ea : Product  Inputs=*/
  Product_09634 : Product
  Product_361a8 : Product
  Product_40c74 : Product
  Product_71e3a : Product
  Product_b0c37 : Product
  Product_b871a : Product
  Product_c812b : Product
  Blockout_d_Px_3_SG_D_1_7e78e : Outport
  wires:
  Constant_T_w_ae441/1 -> Divide_cb6ea/2
  Constant_-1_4b8fe/1 -> Product_b0c37/1
  Add_ae2ce/1 -> Blockout_d_Px_3_SG_D_1_7e78e/1
  Constant_-2.0_88e6c/1 -> Product_361a8/1
  State_w_SG_D_1_3e7b9/1 -> Add_3e2d0/2
  Constant_f0_8479a/1 -> Product_40c74/2
  State_Px_1_SG_D_1_15fdf/1 -> Product_b0c37/2
  Constant_pi_eb74e/1 -> Product_361a8/2
  Product_40c74/1 -> Add_3e2d0/1
  Product_361a8/1 -> Product_40c74/1
  Product_b0c37/1 -> Divide_cb6ea/1
  Divide_63b10/1 -> Add_ae2ce/1
  Constant_T_3_c6588/1 -> Divide_b4ce1/2
  Add_3e2d0/1 -> Divide_2beb5/1
  Constant_T_w_17b7c/1 -> Divide_2beb5/2
  Divide_cb6ea/1 -> Add_5625b/1
  Divide_2beb5/1 -> Add_5625b/2
  Constant_-1_6b6a5/1 -> Product_71e3a/1
  Constant_T_2_9e5a4/1 -> Product_c812b/1
  Add_5625b/1 -> Product_c812b/2
  Constant_-1_78b1b/1 -> Product_09634/1
  Divide_b4ce1/1 -> Add_ae2ce/2
  Constant_T_3_8bbd7/1 -> Divide_63b10/2
  State_Px_2_SG_D_1_a6db1/1 -> Product_09634/2
  State_Px_1_SG_D_1_a9a67/1 -> Add_8be64/1
  Divide_c2e41/1 -> Add_ee9ea/1
  Product_c812b/1 -> Add_8be64/2
  Product_09634/1 -> Divide_c2e41/1
  Product_71e3a/1 -> Divide_63b10/1
  Constant_T_1_cb6f1/1 -> Divide_c2e41/2
  Add_8be64/1 -> Divide_0b283/1
  Constant_T_1_5adde/1 -> Divide_0b283/2
  Divide_0b283/1 -> Add_ee9ea/2
  Constant_T_4_0db6e/1 -> Product_b871a/1
  Add_ee9ea/1 -> Product_b871a/2
  State_Px_3_SG_D_1_17088/1 -> Product_71e3a/2
  State_Px_2_SG_D_1_8d556/1 -> Add_a5a7f/1
  Product_b871a/1 -> Add_a5a7f/2
  Add_a5a7f/1 -> Divide_b4ce1/1

== system IEEE9_case/SG_D_1/d_R_f_SG_D_1_block ==
  note: d_R_f_SG_D_1 in IEEE9_case
      | $-\frac{R_{f,\mathrm{SG},D,1}-\frac{E_{\mathrm{fd},\mathrm{SG},D,1}\,K_{F}}{T_{F}}}{T_{F}}$
      | Automatically generated on 2025-11-01 08:48:02 .
  State_E_fd_SG_D_1_74d9e : Inport
  State_R_f_SG_D_1_1a98f : Inport  Port=2
  Constant_K_F_694ff : Constant  Value=K_F
  Constant_T_F_2524a : Constant  Value=T_F
  Constant_T_F_ef3c9 : Constant  Value=T_F
  Divide_41bc7 : Product  Inputs=*/
  Divide_56837 : Product  Inputs=*/
  Product_dafb5 : Product
  Subtract_8b489 : Sum  Inputs=+-
  Blockout_d_R_f_SG_D_1_506d3 : Outport
  wires:
  Constant_K_F_694ff/1 -> Product_dafb5/2
  Product_dafb5/1 -> Divide_41bc7/1
  State_E_fd_SG_D_1_74d9e/1 -> Product_dafb5/1
  State_R_f_SG_D_1_1a98f/1 -> Subtract_8b489/2
  Constant_T_F_2524a/1 -> Divide_41bc7/2
  Divide_41bc7/1 -> Subtract_8b489/1
  Divide_56837/1 -> Blockout_d_R_f_SG_D_1_506d3/1
  Subtract_8b489/1 -> Divide_56837/1
  Constant_T_F_ef3c9/1 -> Divide_56837/2
